simulink model "ADCS"  (R2020b)
settings: Solver=ode3  StartTime=0.0  StopTime=86400  FixedStep=Ts  RelTol=1e-3
undefined symbols (not defined in the file): Earth, gains, initCond, WGS84
libraries: aerolibutil x9, sharedtransform x4, aerolibconvert2 x3, sharedutil x2, aerolibcubesat x1, pid_lib x1, SignalEditorBlockLib x1, environmentLib x1, aerolib6dof2 x1, asbCubeSatBlockLib x1, aerolibobsolete x1, aerolibattitudesys x1
settings Model: Creator=dbell44  LastModifiedBy=dbell44

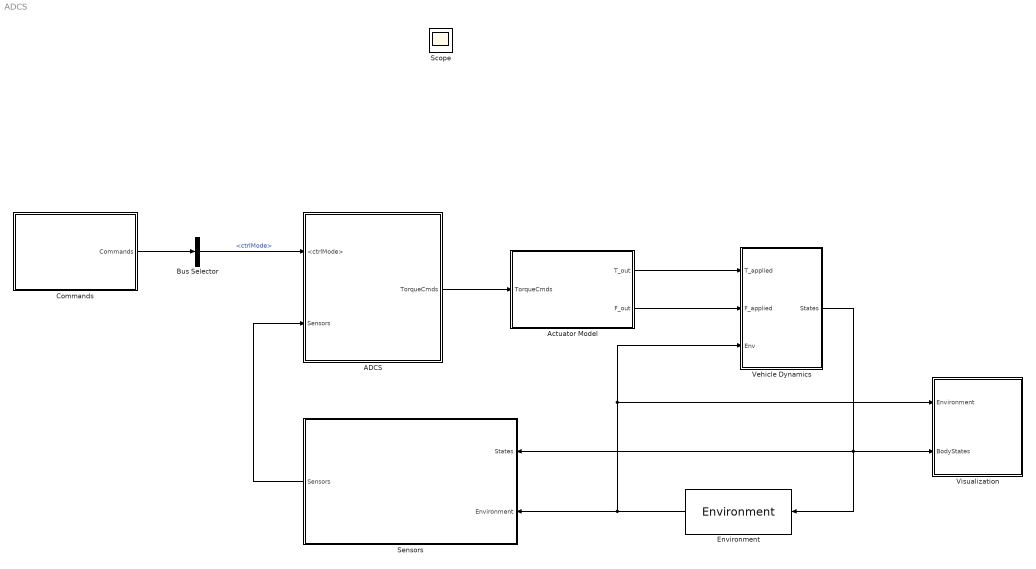
== system ADCS ==
  ADCS : Subsystem
  Actuator Model : Subsystem
  Bus Selector : BusSelector  OutputSignals=ctrlMode
  Commands : Subsystem
  Environment : environmentLib/Environment  SystemSampleTime=-1  VariantActivationTime=update diagram  Latency=0  AutoFrameSizeCalculation=off
  Sensors : Subsystem
  Vehicle Dynamics : Subsystem
  Visualization : Subsystem  Variant=on  mask(Set Animation Properties){visSampleTime=5, cubesatSize=2e5, showAntenna=on, antennaHeight=1e6, antennaHalfAngle=25}
      mask prompts: visSampleTime "aeroblks_cubesat:cubesat:AnimSampleTime"; cubesatSize "aeroblks_cubesat:cubesat:MdlSize"; showAntenna "aeroblks_cubesat:cubesat:ShowCone"; antennaHeight "aeroblks_cubesat:cubesat:ConeHeight"; antennaHalfAngle "aeroblks_cubesat:cubesat:ConeAngle"
      mask help: aeroblks_cubesat:cubesat:VisBlockDesc
      mask Callback showAntenna:
      | if evalin('base', 'exist(''variantVisualization'',''var'')') ...
      |     && evalin('base', 'variantVisualization == 1') ...
      |     && builtin('license','test','Virtual_Reality_Toolbox')
      | 
      |     enable = get_param(gcb,'MaskEnables');
      |     if strcmp(get_param(gcb, 'showAntenna'), 'off')
      |         enable(4:5) = {'off'};
      |     else
      |         enable(4:5) = {'on'};
      |     end
      |     set_param(gcb,'MaskEnables', enable);
      |     clear enable
      | end
      mask DialogControl vrOpenBtn Prompt: aeroblks_cubesat:cubesat:AnimOpenBtn
      mask DialogControl vrOpenBtn Callback:
      | if builtin('license','checkout','Virtual_Reality_Toolbox')
      |     vrmfunc('FnOpen',getSimulinkBlockHandle([gcb '/Virtual Reality World/VR Sink']));
      | end
      mask DialogControl visSampleTime Prompt: Animation refresh rate:
      mask DialogControl visSampleTime Tooltip: aeroblks_cubesat:cubesat:AnimSampleTimeTT
      mask DialogControl cubesatSize Prompt: CubeSat display size [m]:
      mask DialogControl cubesatSize Tooltip: aeroblks_cubesat:cubesat:MdlSizeTT
      mask DialogControl Container3 Prompt: aeroblks_cubesat:cubesat:AntennaPropArea
      mask DialogControl showAntenna Prompt: Show antenna cone in animation
      mask DialogControl showAntenna Tooltip: aeroblks_cubesat:cubesat:ShowConeTT
      mask DialogControl antennaHeight Prompt: Antenna cone height [m]:
      mask DialogControl antennaHeight Tooltip: aeroblks_cubesat:cubesat:ConeHeightTT
      mask DialogControl antennaHalfAngle Prompt: Antenna cone half angle [deg]:
      mask DialogControl antennaHalfAngle Tooltip: aeroblks_cubesat:cubesat:ConeAngleTT
  Scope : Scope
  wires:
  Commands/1(Commands) -> Bus Selector/1
  Environment/1 -> Visualization/1(Environment), Vehicle Dynamics/3(Env), Sensors/2(Environment)
  Bus Selector/1 -> ADCS/1(<ctrlMode>)  "<ctrlMode>"
  Sensors/1(Sensors) -> ADCS/2(Sensors)
  ADCS/1(TorqueCmds) -> Actuator Model/1(TorqueCmds)
  Vehicle Dynamics/1(States) -> Environment/1, Visualization/2(BodyStates), Sensors/1(States)
  Actuator Model/1(T_out) -> Vehicle Dynamics/1(T_applied)
  Actuator Model/2(F_out) -> Vehicle Dynamics/2(F_applied)

== system ADCS/ADCS ==
  <ctrlMode> : Inport
  Sensors : Inport  Port=2
  Attitude Control : Subsystem
  Discrete PID Controller : pid_lib/PID Controller  Controller=PID  Form=Parallel  TimeDomain=Discrete-time  UseExternalTs=off  SampleTime=-1  IntegratorMethod=Forward Euler  FilterMethod=Forward Euler  ControllerParametersSource=internal  P=gains.Kp  I=gains.Ki  D=gains.Kd  UseFilter=off  N=100  TunerSelectOption=Transfer Function Based (PID Tuner App)  InitialConditionSource=internal  InitialConditionForIntegrator=0  InitialConditionForFilter=0  DifferentiatorICPrevScaledInput=0  ExternalReset=none  TrackingMode=off  Kt=1  LimitOutput=off  SatLimitsSource=internal  UpperSaturationLimit=inf  LowerSaturationLimit=-inf  LinearizeAsGain=off  AntiWindupMode=none  Kb=1  POutMin=[]  POutMax=[]  IOutMin=[]  IOutMax=[]  DOutMin=[]  DOutMax=[]  NOutMin=[]  NOutMax=[]  SumOutMin=[]  SumOutMax=[]  SaturationOutMin=[]  SaturationOutMax=[]  PParamMin=[]  PParamMax=[]  IParamMin=[]  IParamMax=[]  DParamMin=[]  DParamMax=[]  NParamMin=[]  NParamMax=[]  KbParamMin=[]  KbParamMax=[]  KtParamMin=[]  KtParamMax=[]  KbOutMin=[]  KbOutMax=[]  KtOutMin=[]  KtOutMax=[]  IntegratorOutMin=[]  IntegratorOutMax=[]  FilterOutMin=[]  FilterOutMax=[]  SumI1OutMin=[]  SumI1OutMax=[]  SumI2OutMin=[]  SumI2OutMax=[]  SumI3OutMin=[]  SumI3OutMax=[]  SumI4OutMin=[]  SumI4OutMax=[]  SumDOutMin=[]  SumDOutMax=[]  DifferentiatorOutMin=[]  DifferentiatorOutMax=[]  FilterDiffOutCoefMin=[]  FilterDiffOutCoefMax=[]  ReciprocalOutMin=[]  ReciprocalOutMax=[]  SumDenOutMin=[]  SumDenOutMax=[]  SumNumOutMin=[]  SumNumOutMax=[]  DivideOutMin=[]  DivideOutMax=[]  UdiffTsProdOutMin=[]  UdiffTsProdOutMax=[]  NTsProdOutMin=[]  NTsProdOutMax=[]  UintegralTsProdOutMin=[]  UintegralTsProdOutMax=[]  UngainTsProdOutMin=[]  UngainTsProdOutMax=[]  IntegratorContinuousStateAttributes=''  IntegratorStateMustResolveToSignalObject=off  IntegratorRTWStateStorageClass=Auto  FilterContinuousStateAttributes=''  FilterStateMustResolveToSignalObject=off  FilterRTWStateStorageClass=Auto  ParallelPVariant=InternalParameters  IdealPVariant=Disabled  IVariant=InternalParameters  DVariant=InternalParameters  IntegratorVariant=Discrete  SatVariant=Disabled  AWVariant=Passthrough  PCopyVariant=Disabled  TRVariant=Disabled  FdbkBlocksVariant=Forward  IdealPFdbkVariant=Disabled  SatFdbkVariant=Disabled  DerivativeFilterVariant=Differentiator  NVariant=Passthrough  NCopyVariant=Disabled_SignalSpec  FilterICVariant=InternalICsDifferentiator  IntegratorICVariant=InternalICs  ExternalResetVariant=Disabled  TRSumVariant=Passthrough  SumFdbkVariant=Disabled  SumVariant=Sum_PID  TsampFilterVariant=InternalTs  TsampNgainVariant=Passthrough  TsampIntegralVariant=Passthrough  ExternalSaturationOutDataTypeStr=Inherit: Same as second input
  Terminator : Terminator
  TorqueCmds : Outport
  wires:
  Sensors/1 -> Attitude Control/1(Sensors)
  Attitude Control/2(ControlMode) -> Terminator/1
  Discrete PID Controller/1 -> TorqueCmds/1
  Attitude Control/1(AttitudeError) -> Discrete PID Controller/1
  <ctrlMode>/1 -> Attitude Control/2(ctrlMode)

== system ADCS/Actuator Model ==
  TorqueCmds : Inport
  Ground : Ground
  T_out : Outport
  F_out : Outport  Port=2
  wires:
  TorqueCmds/1 -> T_out/1
  Ground/1 -> F_out/1

== system ADCS/Commands ==
  Bus Creator : BusCreator  Inputs=2
  Mode : Constant
  Multiport Switch : MultiPortSwitch  DataPortOrder=Specify indices  DataPortIndices={3, [0,1,2]}  DiagnosticForDefault=None
  Signal Editor : SignalEditorBlockLib/Signal Editor  Commented=on  FileName=untitled.mat  ActiveScenario=Scenario  ActiveSignal=Signal 1  IsBus=off  OutputBusObjectStr=Bus: BusObject  SampleTime=0  Interpolate=off  ZeroCross=off  OutputAfterFinalValue=Setting to zero  Unit=inherit  PreserveSignalName=on
  TargetCoords : Constant  Value=[43.26128951472562, -79.90916059630679, 115]
  Commands : Outport
  wires:
  Bus Creator/1 -> Commands/1
  TargetCoords/1 -> Bus Creator/2  "target"
  Multiport Switch/1 -> Bus Creator/1  "ctrlMode"
  Mode/1 -> Multiport Switch/3, Multiport Switch/1
  Signal Editor/1 -> Multiport Switch/2

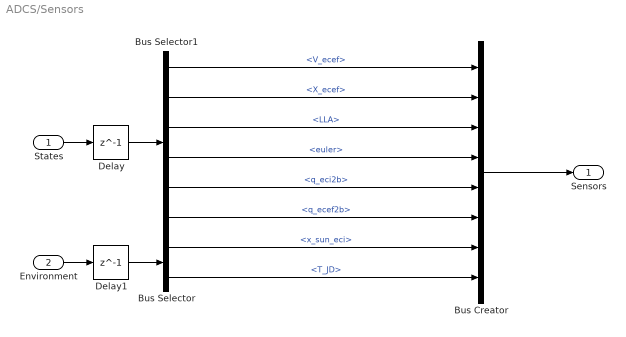
== system ADCS/Sensors ==
  States : Inport  OutDataTypeStr=Bus: States
  Environment : Inport  Port=2
  Bus Creator : BusCreator  Inputs=8
  Bus Selector : BusSelector  OutputSignals=x_sun_eci,T_JD
  Bus Selector1 : BusSelector  OutputSignals=V_ecef,X_ecef,LLA,euler,q_eci2b,q_ecef2b
  Delay : Delay  DelayLength=1  InitialCondition=0
  Delay1 : Delay  DelayLength=1  InitialCondition=0
  Sensors : Outport
  wires:
  Environment/1 -> Delay1/1
  Bus Selector/1 -> Bus Creator/7  "<x_sun_eci>"
  Bus Selector/2 -> Bus Creator/8  "<T_JD>"
  States/1 -> Delay/1
  Bus Creator/1 -> Sensors/1
  Bus Selector1/1 -> Bus Creator/1  "<V_ecef>"
  Bus Selector1/2 -> Bus Creator/2  "<X_ecef>"
  Bus Selector1/3 -> Bus Creator/3  "<LLA>"
  Bus Selector1/4 -> Bus Creator/4  "<euler>"
  Bus Selector1/5 -> Bus Creator/5  "<q_eci2b>"
  Bus Selector1/6 -> Bus Creator/6  "<q_ecef2b>"
  Delay/1 -> Bus Selector1/1
  Delay1/1 -> Bus Selector/1

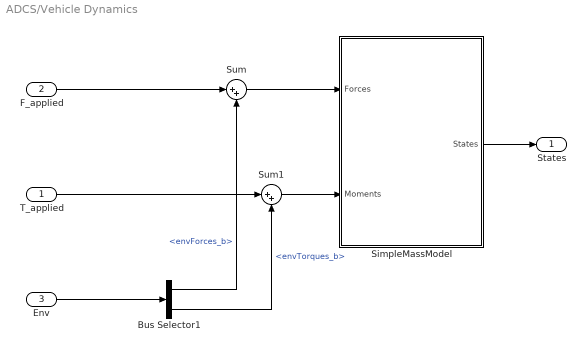
== system ADCS/Vehicle Dynamics ==
  T_applied : Inport
  F_applied : Inport  Port=2
  Env : Inport  Port=3
  Bus Selector1 : BusSelector  OutputSignals=envForces_b,envTorques_b
  SimpleMassModel : Subsystem
  Sum : Sum  Inputs=|++
  Sum1 : Sum  Inputs=|++
  States : Outport  OutDataTypeStr=Bus: States
  wires:
  Sum/1 -> SimpleMassModel/1(Forces)
  Bus Selector1/1 -> Sum/2  "<envForces_b>"
  T_applied/1 -> Sum1/1
  F_applied/1 -> Sum/1
  Bus Selector1/2 -> Sum1/2  "<envTorques_b>"
  SimpleMassModel/1(States) -> States/1
  Env/1 -> Bus Selector1/1
  Sum1/1 -> SimpleMassModel/2(Moments)

== system ADCS/Visualization ==
  Environment : Inport
  BodyStates : Inport  Port=2
  No Visualization : Subsystem  VariantControl=visOff
  Virtual Reality World : Subsystem  VariantControl=visSL3D

== system ADCS/ADCS/Attitude Control ==
  Sensors : Inport
  ctrlMode : Inport  Port=2
  Control Mode Selector : Stateflow chart  TreatAsAtomicUnit=on
  AttitudeError : Outport
  ControlMode : Outport  Port=2
  wires:
  Sensors/1 -> Control Mode Selector/1(Sensors)
  ctrlMode/1 -> Control Mode Selector/2(ctrlMode)
  Control Mode Selector/1(AttitudeError) -> AttitudeError/1
  Control Mode Selector/2(ControlMode) -> ControlMode/1

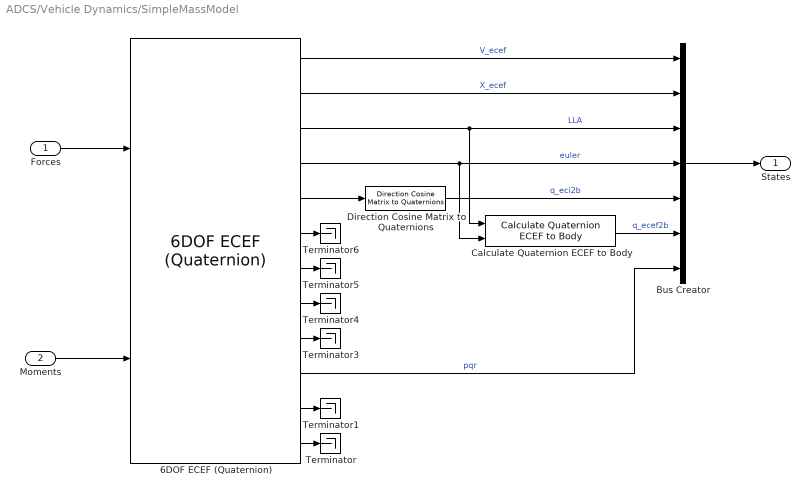
== system ADCS/Vehicle Dynamics/SimpleMassModel ==
  Forces : Inport
  Moments : Inport  Port=2
  6DOF ECEF (Quaternion) : aerolib6dof2/6DOF ECEF (Quaternion)  units=Metric (MKS)  mtype=Fixed  xg_0=initCond.lla  Vm_0=initCond.uvw  eul_0=deg2rad(initCond.euler)  pm_0=deg2rad(initCond.pqr)  mass_0=vehicle.mass  mass_e=0.5  mass_f=2.0  inertia=vehicle.inertia  inertia_e=eye(3)  inertia_f=2*eye(3)  vre_flag=on  abi_flag=off  ptype=Earth (WGS84)  R=6378137  F=1/298.257223563  w_E=7292115e-11  angle_in=Internal  LG0=initCond.EarthProps.LG  quat_statename=''  pm_statename=''  Vm_statename=''  posECEF_statename=''  posECI_statename=''  LG_statename=''  mass_statename=''
      settings: SourceProductBaseCode=AE
  Bus Creator : BusCreator  Inputs=7  OutDataTypeStr=Bus: States
      settings: InheritFromInputs=off
  Calculate Quaternion ECEF to Body : asbCubeSatBlockLib/Axes Transformations/Coordinate System Transformations/Calculate Quaternion ECEF to Body  SystemSampleTime=-1  VariantActivationTime=update diagram  Latency=0  AutoFrameSizeCalculation=off
      settings: SourceProductBaseCode=AERO_CUBESAT
  Direction Cosine Matrix to Quaternions : sharedtransform/Direction Cosine Matrix  to Quaternions  aMode=0  action=None  tolerance=eps(2)
      settings: SourceProductBaseCode=AE,PW,MT,UV,VE,VP
  Terminator{,1,3..6} (6 alike) : Terminator
  States : Outport  OutDataTypeStr=Bus: States
  wires:
  6DOF ECEF (Quaternion)/12 -> Terminator/1
  Calculate Quaternion ECEF to Body/1 -> Bus Creator/6  "q_ecef2b"
  Forces/1 -> 6DOF ECEF (Quaternion)/1
  6DOF ECEF (Quaternion)/11 -> Terminator1/1
  6DOF ECEF (Quaternion)/4 -> Bus Creator/4, Calculate Quaternion ECEF to Body/2  "euler"
  Moments/1 -> 6DOF ECEF (Quaternion)/2
  6DOF ECEF (Quaternion)/6 -> Terminator6/1
  6DOF ECEF (Quaternion)/8 -> Terminator4/1
  6DOF ECEF (Quaternion)/5 -> Direction Cosine Matrix to Quaternions/1
  6DOF ECEF (Quaternion)/1 -> Bus Creator/1  "V_ecef"
  Direction Cosine Matrix to Quaternions/1 -> Bus Creator/5  "q_eci2b"
  6DOF ECEF (Quaternion)/10 -> Bus Creator/7  "pqr"
  6DOF ECEF (Quaternion)/2 -> Bus Creator/2  "X_ecef"
  6DOF ECEF (Quaternion)/9 -> Terminator3/1
  Bus Creator/1 -> States/1
  6DOF ECEF (Quaternion)/7 -> Terminator5/1
  6DOF ECEF (Quaternion)/3 -> Bus Creator/3, Calculate Quaternion ECEF to Body/1  "LLA"

== system ADCS/Visualization/No Visualization ==
  BodyStates : Inport
  Environment : Inport  Port=2
  Terminator2 : Terminator
  Terminator3 : Terminator
  wires:
  Environment/1 -> Terminator2/1
  BodyStates/1 -> Terminator3/1

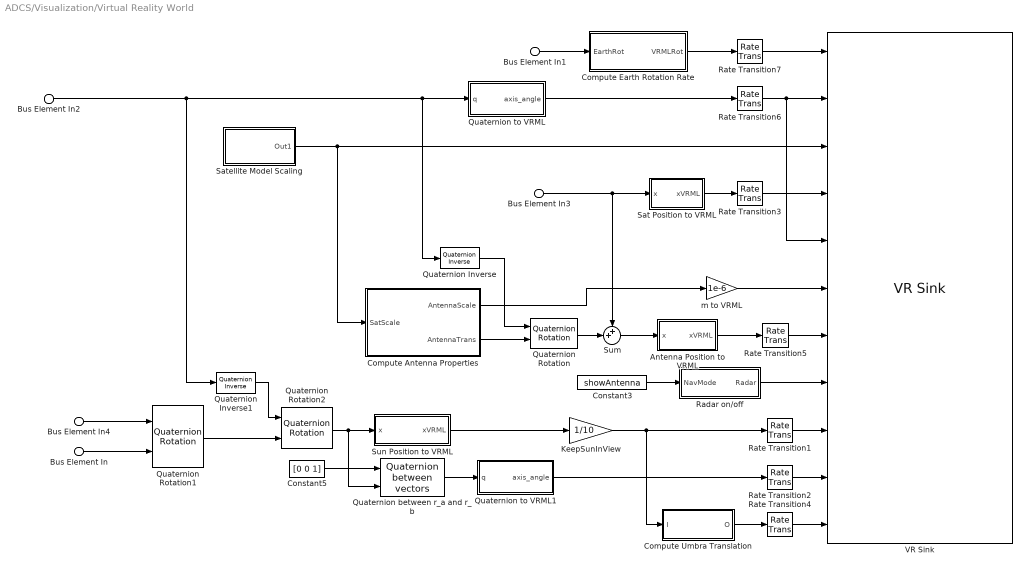
== system ADCS/Visualization/Virtual Reality World ==
  Bus Element In3 : Inport  PortName=BodyStates  Element=X_ecef
  Bus Element In2 : Inport  PortName=BodyStates  Element=q_ecef2b
  Bus Element In4 : Inport  PortName=BodyStates  Element=q_eci2b
  Bus Element In : Inport  Port=2  PortName=Environment  Element=x_sun_eci
  Bus Element In1 : Inport  Port=2  PortName=Environment  Element=earthAngRate
  Antenna Position to VRML : Subsystem
  Compute Antenna Properties : Subsystem
  Compute Earth Rotation Rate : Subsystem
  Compute Umbra Translation : Subsystem
  Constant3 : Constant  Value=showAntenna
  Constant5 : Constant  Value=[0 0 1]
  KeepSunInView : Gain  Gain=1/10
  Quaternion Inverse : aerolibutil/Quaternion Inverse
      settings: SourceProductName=Aerospace Blockset
  Quaternion Inverse1 : aerolibutil/Quaternion Inverse
      settings: SourceProductName=Aerospace Blockset
  Quaternion Rotation : aerolibutil/Quaternion Rotation
  Quaternion Rotation1 : aerolibutil/Quaternion Rotation
  Quaternion Rotation2 : aerolibutil/Quaternion Rotation
  Quaternion between r_a and r_b : aerolibattitudesys/Quaternion between vectors
      settings: SourceProductBaseCode=AERO_CUBESAT
  Quaternion to VRML : Subsystem
  Quaternion to VRML1 : Subsystem
  Radar on/off : Subsystem
  Rate Transition{1..7} (7 alike) : RateTransition
  Sat Position to VRML : Subsystem
  Satellite Model Scaling : Subsystem
  Sum : Sum  Inputs=++|
  Sun Position to VRML : Subsystem
  VR Sink : vrlib/VR Sink  InstantiateOnLoad=on  SampleTime=visSampleTime  ViewEnable=on  RemoteChange=off  RemoteView=off  FieldsWritten=Earth.rotation.4.1.1.double#Satellite.rotation.4.1.1.double#Satellite.scale.3.1.1.double#Satellite.translation.3.1.1.double#AntennaCone.rotation.4.1.1.double#AntennaCone.scale.3.1.1.double#AntennaCone.translation.3.1.1.double#AntennaMaterial.transparency.1.1.1.double#Sun.translation.3.1.1.double#Umbra.rotation.4.1.1.double#Umbra.translation.3.1.1.double  WorldFileName=cubesatAnim.wrl  WorldDescription=CubeSat Orbit Animation  AutoView=on  VideoDimensions=[]  AllowVariableSize=off
  m to VRML : Gain  Gain=1e-6
  wires:
  Bus Element In2/1 -> Quaternion to VRML/1(q), Quaternion Inverse/1, Quaternion Inverse1/1
  Constant3/1 -> Radar on/off/1(NavMode)
  Bus Element In3/1 -> Sat Position to VRML/1(x), Sum/1
  Quaternion Inverse/1 -> Quaternion Rotation/1
  Sum/1 -> Antenna Position to VRML/1(x)
  Quaternion Rotation/1 -> Sum/2
  Quaternion Rotation2/1 -> Sun Position to VRML/1(x), Quaternion between r_a and r_b/2
  Quaternion Rotation1/1 -> Quaternion Rotation2/2
  Quaternion Inverse1/1 -> Quaternion Rotation2/1
  Sun Position to VRML/1(xVRML) -> KeepSunInView/1
  Quaternion between r_a and r_b/1 -> Quaternion to VRML1/1(q)
  Constant5/1 -> Quaternion between r_a and r_b/1
  m to VRML/1 -> VR Sink/6
  Antenna Position to VRML/1(xVRML) -> Rate Transition5/1
  Compute Earth Rotation Rate/1(VRMLRot) -> Rate Transition7/1
  Sat Position to VRML/1(xVRML) -> Rate Transition3/1
  Radar on/off/1(Radar) -> VR Sink/8
  Quaternion to VRML1/1(axis_angle) -> Rate Transition2/1
  KeepSunInView/1 -> Compute Umbra Translation/1(I), Rate Transition1/1
  Compute Umbra Translation/1(O) -> Rate Transition4/1
  Satellite Model Scaling/1(Out1) -> VR Sink/3, Compute Antenna Properties/1(SatScale)
  Compute Antenna Properties/1(AntennaScale) -> m to VRML/1
  Compute Antenna Properties/2(AntennaTrans) -> Quaternion Rotation/2
  Bus Element In4/1 -> Quaternion Rotation1/1
  Bus Element In/1 -> Quaternion Rotation1/2
  Rate Transition4/1 -> VR Sink/11
  Rate Transition1/1 -> VR Sink/9
  Rate Transition2/1 -> VR Sink/10
  Bus Element In1/1 -> Compute Earth Rotation Rate/1(EarthRot)
  Rate Transition7/1 -> VR Sink/1
  Rate Transition3/1 -> VR Sink/4
  Rate Transition5/1 -> VR Sink/7
  Quaternion to VRML/1(axis_angle) -> Rate Transition6/1
  Rate Transition6/1 -> VR Sink/5, VR Sink/2

== system ADCS/ADCS/Attitude Control/Control Mode Selector/Off ==
  " " : ActionPort
      settings: CopyFcn=Stateflow.SLINSF.SimulinkMan.removeBlockPreDeleteFcn  PreDeleteFcn=Stateflow.SLINSF.SimulinkMan.unsafePredeleteFcn
  ActuatorsOff : Constant  Value=[0 0 0]
  AttitudeError : Outport
  wires:
  ActuatorsOff/1 -> AttitudeError/1  "torque_cmd"

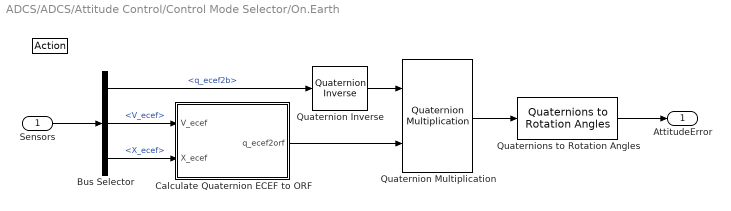
== system ADCS/ADCS/Attitude Control/Control Mode Selector/On.Earth ==
  Sensors : Inport
  " " : ActionPort
      settings: CopyFcn=Stateflow.SLINSF.SimulinkMan.removeBlockPreDeleteFcn  PreDeleteFcn=Stateflow.SLINSF.SimulinkMan.unsafePredeleteFcn
  Bus Selector : BusSelector  OutputSignals=q_ecef2b,V_ecef,X_ecef
  Calculate Quaternion ECEF to ORF : Subsystem
  Quaternion Inverse : aerolibutil/Quaternion Inverse
      settings: SourceProductName=Aerospace Blockset
  Quaternion Multiplication : aerolibutil/Quaternion Multiplication
  Quaternions to Rotation Angles : sharedtransform/Quaternions to Rotation Angles  rotationOrder=XYZ  aMode=aMode
      settings: SourceProductBaseCode=AE,PW,MT,UV,VE,VP
  AttitudeError : Outport  VectorParamsAs1DForOutWhenUnconnected=off
  wires:
  Quaternions to Rotation Angles/1 -> AttitudeError/1
  Quaternion Inverse/1 -> Quaternion Multiplication/1
  Quaternion Multiplication/1 -> Quaternions to Rotation Angles/1
  Calculate Quaternion ECEF to ORF/1(q_ecef2orf) -> Quaternion Multiplication/2
  Bus Selector/1 -> Quaternion Inverse/1  "<q_ecef2b>"
  Bus Selector/3 -> Calculate Quaternion ECEF to ORF/2(X_ecef)  "<X_ecef>"
  Bus Selector/2 -> Calculate Quaternion ECEF to ORF/1(V_ecef)  "<V_ecef>"
  Sensors/1 -> Bus Selector/1

== system ADCS/ADCS/Attitude Control/Control Mode Selector/On.Sun ==
  Sensors : Inport
  " " : ActionPort
      settings: CopyFcn=Stateflow.SLINSF.SimulinkMan.removeBlockPreDeleteFcn  PreDeleteFcn=Stateflow.SLINSF.SimulinkMan.unsafePredeleteFcn
  Attitude Profile : aerolibcubesat/Spacecraft Dynamics/Attitude Profile  portFrame=Fixed-frame  pointingMode=Point at celestial body  celestialTarget=Sun  tunablePointing=off  primaryAlignmentSrc=Dialog  primaryAlignment=[0 0 1]  secondaryAlignmentSrc=Dialog  secondaryAlignment=[1 0 0]  constraintFrame=LVLH  primaryConstraintSrc=Dialog  primaryConstraint=[1 0 0]  secondaryConstraintSrc=Dialog  secondaryConstraint=[0 1 0]
      settings: AttributesFormatString=%<pointingMode>  SourceProductBaseCode=AERO_CUBESAT
  Bus Selector : BusSelector  OutputSignals=T_JD,X_ecef,V_ecef,q_ecef2b
  Quaternions to Rotation Angles : sharedtransform/Quaternions to Rotation Angles  rotationOrder=XYZ  aMode=aMode
      settings: SourceProductBaseCode=AE,PW,MT,UV,VE,VP
  AttitudeError : Outport
  wires:
  Sensors/1 -> Bus Selector/1
  Bus Selector/1 -> Attitude Profile/1  "<T_JD>"
  Bus Selector/3 -> Attitude Profile/3  "<V_ecef>"
  Bus Selector/2 -> Attitude Profile/2  "<X_ecef>"
  Bus Selector/4 -> Attitude Profile/4  "<q_ecef2b>"
  Attitude Profile/1 -> Quaternions to Rotation Angles/1
  Quaternions to Rotation Angles/1 -> AttitudeError/1

== system ADCS/Visualization/Virtual Reality World/Antenna Position to VRML ==
  x : Inport
  ECEF to VRML : Subsystem
  Length Conversion : aerolibconvert2/Length Conversion  IU=m  OU=km
  km to VRML units : Gain  Gain=1/1000
  xVRML : Outport  VectorParamsAs1DForOutWhenUnconnected=off
  wires:
  Length Conversion/1 -> km to VRML units/1
  km to VRML units/1 -> ECEF to VRML/1(M)
  x/1 -> Length Conversion/1
  ECEF to VRML/1(VR) -> xVRML/1

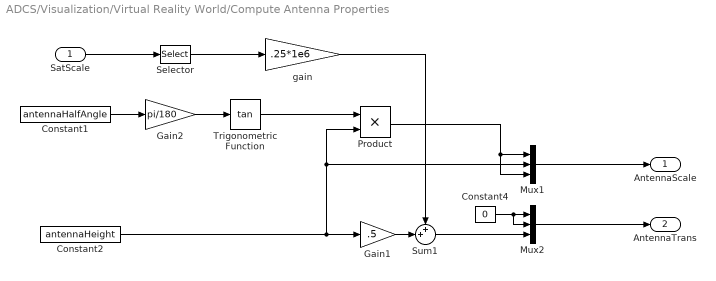
== system ADCS/Visualization/Virtual Reality World/Compute Antenna Properties ==
  SatScale : Inport
  Constant1 : Constant  Value=antennaHalfAngle
  Constant2 : Constant  Value=antennaHeight
  Constant4 : Constant  Value=0
  Gain1 : Gain  Gain=.5
  Gain2 : Gain  Gain=pi/180
  Mux1 : Mux  Inputs=3
  Mux2 : Mux  Inputs=3
  Product : Product
  Selector : Selector  InputPortWidth=3  IndexOptions=Index vector (dialog)  Indices=1  OutputSizes=1
  Sum1 : Sum  Inputs=++|
  Trigonometric Function : Trigonometry  Operator=tan
  gain : Gain  Gain=.25*1e6
  AntennaScale : Outport  VectorParamsAs1DForOutWhenUnconnected=off
  AntennaTrans : Outport  Port=2  VectorParamsAs1DForOutWhenUnconnected=off
  wires:
  Gain2/1 -> Trigonometric Function/1
  Constant4/1 -> Mux2/1, Mux2/2
  Sum1/1 -> Mux2/3
  Constant2/1 -> Gain1/1, Mux1/2, Product/2
  gain/1 -> Sum1/1
  Constant1/1 -> Gain2/1
  Product/1 -> Mux1/3, Mux1/1
  Gain1/1 -> Sum1/2
  Trigonometric Function/1 -> Product/1
  Mux2/1 -> AntennaTrans/1
  Mux1/1 -> AntennaScale/1
  SatScale/1 -> Selector/1
  Selector/1 -> gain/1

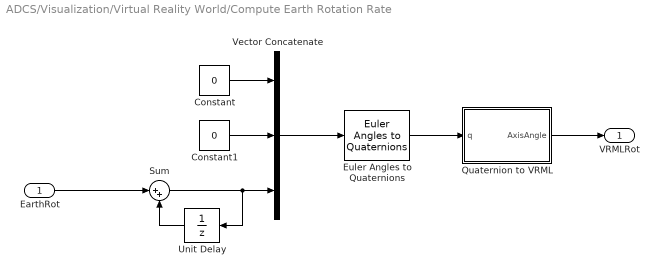
== system ADCS/Visualization/Virtual Reality World/Compute Earth Rotation Rate ==
  EarthRot : Inport
  Constant : Constant  Value=0
  Constant1 : Constant  Value=0
  Euler Angles to Quaternions : aerolibobsolete/Euler Angles to Quaternions
      settings: SourceProductBaseCode=AE
  Quaternion to VRML : Subsystem
  Sum : Sum  Inputs=|++
  Unit Delay : UnitDelay  SampleTime=-1  HasFrameUpgradeWarning=on
  Vector Concatenate : Concatenate  NumInputs=3
  VRMLRot : Outport  VectorParamsAs1DForOutWhenUnconnected=off
  wires:
  EarthRot/1 -> Sum/1
  Unit Delay/1 -> Sum/2
  Sum/1 -> Vector Concatenate/3, Unit Delay/1
  Constant/1 -> Vector Concatenate/1
  Constant1/1 -> Vector Concatenate/2
  Vector Concatenate/1 -> Euler Angles to Quaternions/1
  Euler Angles to Quaternions/1 -> Quaternion to VRML/1(q)
  Quaternion to VRML/1(AxisAngle) -> VRMLRot/1

== system ADCS/Visualization/Virtual Reality World/Compute Umbra Translation ==
  I : Inport
  Add : Sum
  ConeHalfLength : Gain  Gain=692
  InvertSunPosECEF : Gain  Gain=-1
  unitVec : Subsystem
  O : Outport  VectorParamsAs1DForOutWhenUnconnected=off
  wires:
  ConeHalfLength/1 -> Add/2
  I/1 -> InvertSunPosECEF/1
  Add/1 -> O/1
  InvertSunPosECEF/1 -> unitVec/1(I), Add/1
  unitVec/1(O) -> ConeHalfLength/1

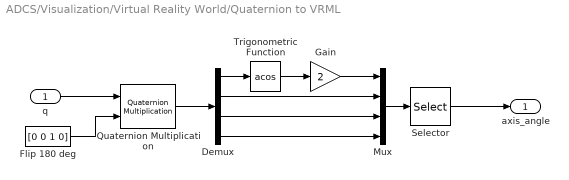
== system ADCS/Visualization/Virtual Reality World/Quaternion to VRML ==
  q : Inport
  Demux : Demux
  Flip 180 deg : Constant  Value=[0 0 1 0]
  Gain : Gain  Gain=2
  Mux : Mux
  Quaternion Multiplication : aerolibutil/Quaternion Multiplication
  Selector : Selector  InputPortWidth=4  IndexOptions=Index vector (dialog)  Indices=[3 4 2 1]  OutputSizes=1
  Trigonometric Function : Trigonometry  Operator=acos
  axis_angle : Outport  VectorParamsAs1DForOutWhenUnconnected=off
  wires:
  Demux/4 -> Mux/4
  Demux/3 -> Mux/3
  Demux/2 -> Mux/2
  Gain/1 -> Mux/1
  Selector/1 -> axis_angle/1
  q/1 -> Quaternion Multiplication/1
  Mux/1 -> Selector/1
  Trigonometric Function/1 -> Gain/1
  Demux/1 -> Trigonometric Function/1
  Flip 180 deg/1 -> Quaternion Multiplication/2
  Quaternion Multiplication/1 -> Demux/1

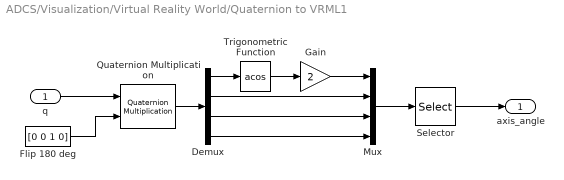
== system ADCS/Visualization/Virtual Reality World/Quaternion to VRML1 ==
  q : Inport
  Demux : Demux
  Flip 180 deg : Constant  Value=[0 0 1 0]
  Gain : Gain  Gain=2
  Mux : Mux
  Quaternion Multiplication : aerolibutil/Quaternion Multiplication
  Selector : Selector  InputPortWidth=4  IndexOptions=Index vector (dialog)  Indices=[3 4 2 1]  OutputSizes=1
  Trigonometric Function : Trigonometry  Operator=acos
  axis_angle : Outport  VectorParamsAs1DForOutWhenUnconnected=off
  wires:
  Demux/4 -> Mux/4
  Demux/3 -> Mux/3
  Demux/2 -> Mux/2
  Gain/1 -> Mux/1
  Selector/1 -> axis_angle/1
  Mux/1 -> Selector/1
  Trigonometric Function/1 -> Gain/1
  Demux/1 -> Trigonometric Function/1
  Flip 180 deg/1 -> Quaternion Multiplication/2
  q/1 -> Quaternion Multiplication/1
  Quaternion Multiplication/1 -> Demux/1

== system ADCS/Visualization/Virtual Reality World/Radar on//off ==
  NavMode : Inport
  Add : Sum  Inputs=-+
  Compare To Constant : simulink/Logic and Bit Operations/Compare To Constant  relop===  const=1  OutDataTypeStr=boolean  ZeroCross=off
  Constant : Constant
  Data Type Conversion : DataTypeConversion  OutDataTypeStr=double
  Gain : Gain  Gain=0.6
  Radar : Outport  VectorParamsAs1DForOutWhenUnconnected=off
  wires:
  NavMode/1 -> Compare To Constant/1
  Compare To Constant/1 -> Data Type Conversion/1
  Data Type Conversion/1 -> Gain/1
  Gain/1 -> Add/1
  Constant/1 -> Add/2
  Add/1 -> Radar/1

== system ADCS/Visualization/Virtual Reality World/Sat Position to VRML ==
  x : Inport
  ECEF to VRML : Subsystem
  Length Conversion : aerolibconvert2/Length Conversion  IU=m  OU=km
  km to VRML units : Gain  Gain=1/1000
  xVRML : Outport  VectorParamsAs1DForOutWhenUnconnected=off
  wires:
  ECEF to VRML/1(VR) -> xVRML/1
  x/1 -> Length Conversion/1
  km to VRML units/1 -> ECEF to VRML/1(M)
  Length Conversion/1 -> km to VRML units/1

== system ADCS/Visualization/Virtual Reality World/Satellite Model Scaling ==
  Constant : Constant  Value=cubesatSize
  Mux : Mux  Inputs=3
  ScaleModelToVRML : Gain  Gain=1/.3e6
  Out1 : Outport  VectorParamsAs1DForOutWhenUnconnected=off
  wires:
  ScaleModelToVRML/1 -> Mux/3, Mux/1, Mux/2
  Constant/1 -> ScaleModelToVRML/1
  Mux/1 -> Out1/1

== system ADCS/Visualization/Virtual Reality World/Sun Position to VRML ==
  x : Inport
  ECEF to VRML : Subsystem
  Length Conversion : aerolibconvert2/Length Conversion  IU=m  OU=km
  km to VRML units : Gain  Gain=1/1000
  xVRML : Outport  VectorParamsAs1DForOutWhenUnconnected=off
  wires:
  ECEF to VRML/1(VR) -> xVRML/1
  x/1 -> Length Conversion/1
  km to VRML units/1 -> ECEF to VRML/1(M)
  Length Conversion/1 -> km to VRML units/1

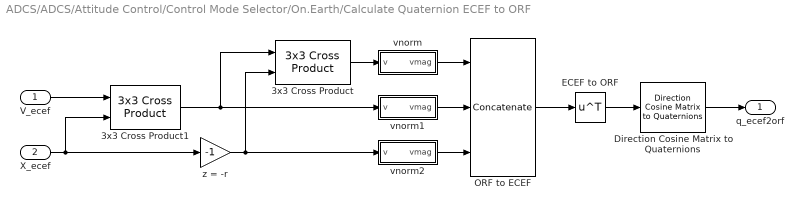
== system ADCS/ADCS/Attitude Control/Control Mode Selector/On.Earth/Calculate Quaternion ECEF to ORF ==
  V_ecef : Inport
  X_ecef : Inport  Port=2
  3x3 Cross Product : sharedutil/3x3 Cross Product  aMode=aMode
      settings: SourceProductBaseCode=AE,PW,MT,UV,VE,VP
  3x3 Cross Product1 : sharedutil/3x3 Cross Product  aMode=aMode
      settings: SourceProductBaseCode=AE,PW,MT,UV,VE,VP
  Direction Cosine Matrix to Quaternions : sharedtransform/Direction Cosine Matrix  to Quaternions  aMode=0  action=None  tolerance=eps(2)
      settings: SourceProductBaseCode=AE,PW,MT,UV,VE,VP
  ECEF to ORF : Math  Operator=transpose  SignedPower=on  SaturateOnIntegerOverflow=on
  ORF to ECEF : Concatenate  NumInputs=3  Mode=Multidimensional array  ConcatenateDimension=2
  vnorm : Subsystem
      mask Display: disp('v norm')
  vnorm1 : Subsystem
      mask Display: disp('v norm')
  vnorm2 : Subsystem
      mask Display: disp('v norm')
  z = -r : Gain  Gain=-1
  q_ecef2orf : Outport  VectorParamsAs1DForOutWhenUnconnected=off
  wires:
  Direction Cosine Matrix to Quaternions/1 -> q_ecef2orf/1
  3x3 Cross Product1/1 -> 3x3 Cross Product/1, vnorm1/1(v)
  X_ecef/1 -> 3x3 Cross Product1/2, z = -r/1
  3x3 Cross Product/1 -> vnorm/1(v)
  z = -r/1 -> 3x3 Cross Product/2, vnorm2/1(v)
  V_ecef/1 -> 3x3 Cross Product1/1
  vnorm1/1(vmag) -> ORF to ECEF/2
  vnorm2/1(vmag) -> ORF to ECEF/3
  vnorm/1(vmag) -> ORF to ECEF/1
  ORF to ECEF/1 -> ECEF to ORF/1
  ECEF to ORF/1 -> Direction Cosine Matrix to Quaternions/1

== system ADCS/Visualization/Virtual Reality World/Antenna Position to VRML/ECEF to VRML ==
  M : Inport  PortDimensions=3
  Selector : Selector  InputPortWidth=3  IndexOptions=Index vector (dialog)  Indices=[2 3 1]  OutputSizes=1
  VR : Outport  PortDimensions=3  VectorParamsAs1DForOutWhenUnconnected=off
  wires:
  M/1 -> Selector/1
  Selector/1 -> VR/1

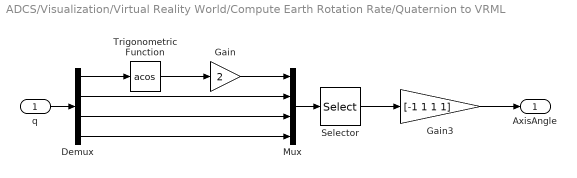
== system ADCS/Visualization/Virtual Reality World/Compute Earth Rotation Rate/Quaternion to VRML ==
  q : Inport
  Demux : Demux
  Gain : Gain  Gain=2
  Gain3 : Gain  Gain=[-1 1 1 1]
  Mux : Mux
  Selector : Selector  InputPortWidth=4  IndexOptions=Index vector (dialog)  Indices=[2 4 3 1]  OutputSizes=1
  Trigonometric Function : Trigonometry  Operator=acos
  AxisAngle : Outport  VectorParamsAs1DForOutWhenUnconnected=off
  wires:
  Demux/4 -> Mux/4
  Demux/3 -> Mux/3
  Demux/2 -> Mux/2
  Gain/1 -> Mux/1
  Selector/1 -> Gain3/1
  Gain3/1 -> AxisAngle/1
  q/1 -> Demux/1
  Mux/1 -> Selector/1
  Trigonometric Function/1 -> Gain/1
  Demux/1 -> Trigonometric Function/1

== system ADCS/Visualization/Virtual Reality World/Compute Umbra Translation/unitVec ==
  I : Inport
  Divide : Product  Inputs=*/
  Dot Product : DotProduct  InputSameDT=on  OutDataTypeStr=Inherit: Inherit via internal rule
  Sqrt : Sqrt  SaturateOnIntegerOverflow=on
  O : Outport  VectorParamsAs1DForOutWhenUnconnected=off
  wires:
  Dot Product/1 -> Sqrt/1
  I/1 -> Divide/1, Dot Product/1, Dot Product/2
  Divide/1 -> O/1
  Sqrt/1 -> Divide/2

== system ADCS/Visualization/Virtual Reality World/Sat Position to VRML/ECEF to VRML ==
  M : Inport  PortDimensions=3
  Selector : Selector  InputPortWidth=3  IndexOptions=Index vector (dialog)  Indices=[2 3 1]  OutputSizes=1
  VR : Outport  PortDimensions=3  VectorParamsAs1DForOutWhenUnconnected=off
  wires:
  M/1 -> Selector/1
  Selector/1 -> VR/1

== system ADCS/Visualization/Virtual Reality World/Sun Position to VRML/ECEF to VRML ==
  M : Inport  PortDimensions=3
  Selector : Selector  InputPortWidth=3  IndexOptions=Index vector (dialog)  Indices=[2 3 1]  OutputSizes=1
  VR : Outport  PortDimensions=3  VectorParamsAs1DForOutWhenUnconnected=off
  wires:
  M/1 -> Selector/1
  Selector/1 -> VR/1

== system ADCS/ADCS/Attitude Control/Control Mode Selector/On.Earth/Calculate Quaternion ECEF to ORF/vnorm ==
  v : Inport
  Divide : Product  Inputs=*/
  Dot Product : DotProduct  InputSameDT=on  OutDataTypeStr=Inherit: Inherit via internal rule
  Math Function1 : Math  Operator=sqrt  SignedPower=on  SaturateOnIntegerOverflow=on
  Sum of Elements : Sum  Inputs=+
  vmag : Outport  VectorParamsAs1DForOutWhenUnconnected=off
  wires:
  Dot Product/1 -> Sum of Elements/1
  Sum of Elements/1 -> Math Function1/1
  Math Function1/1 -> Divide/2
  v/1 -> Divide/1, Dot Product/2, Dot Product/1
  Divide/1 -> vmag/1

== system ADCS/ADCS/Attitude Control/Control Mode Selector/On.Earth/Calculate Quaternion ECEF to ORF/vnorm1 ==
  v : Inport
  Divide : Product  Inputs=*/
  Dot Product : DotProduct  InputSameDT=on  OutDataTypeStr=Inherit: Inherit via internal rule
  Math Function1 : Math  Operator=sqrt  SignedPower=on  SaturateOnIntegerOverflow=on
  Sum of Elements : Sum  Inputs=+
  vmag : Outport  VectorParamsAs1DForOutWhenUnconnected=off
  wires:
  Divide/1 -> vmag/1
  v/1 -> Dot Product/1, Dot Product/2, Divide/1
  Math Function1/1 -> Divide/2
  Sum of Elements/1 -> Math Function1/1
  Dot Product/1 -> Sum of Elements/1

== system ADCS/ADCS/Attitude Control/Control Mode Selector/On.Earth/Calculate Quaternion ECEF to ORF/vnorm2 ==
  v : Inport
  Divide : Product  Inputs=*/
  Dot Product : DotProduct  InputSameDT=on  OutDataTypeStr=Inherit: Inherit via internal rule
  Math Function1 : Math  Operator=sqrt  SignedPower=on  SaturateOnIntegerOverflow=on
  Sum of Elements : Sum  Inputs=+
  vmag : Outport  VectorParamsAs1DForOutWhenUnconnected=off
  wires:
  Dot Product/1 -> Sum of Elements/1
  Sum of Elements/1 -> Math Function1/1
  Math Function1/1 -> Divide/2
  v/1 -> Divide/1, Dot Product/2, Dot Product/1
  Divide/1 -> vmag/1

== stateflow chart ADCS/Attitude Control/Control Mode Selector ==
  settings: updateMethod=DISCRETE  sampleTime=Ts
  state On
    state Transition
    state Earth
    state Sun
    (default) -> Transition
    Transition -> Sun [order 2] : [ctrlMode == 2]
        | {ControlMode = 2;}
    Sun -> Transition : [ctrlMode == 1]
        | {ControlMode = 1;}
    Transition -> Earth [order 1] : [ctrlMode == 1]
        | {ControlMode = 2;}
    Earth -> Transition : [ctrlMode == 2]
        | {ControlMode = 1;}
  state Off
  (default) -> Off
  Off -> On : [ctrlMode ~= 0]
      | {ControlMode = 1;}
  On -> Off : [ctrlMode == 0]
      | {ControlMode = 0;}
  data: sf_internal_action_state_placeholder_data local double size=1 =0; sf_internal_action_state_placeholder_data local double size=1 =0; sf_internal_action_state_placeholder_data local double size=1 =0; Sensors input; ctrlMode input; AttitudeError output =[0 0 0]'; ControlMode output
